simulink model "steeringControlSystemNoFilter"  (R2023b)
settings: Solver=ode4  StartTime=0.0  StopTime=5  FixedStep=0.002  RelTol=1e-3  AbsTol=1e-6  EnableMultiTasking=on
undefined symbols (not defined in the file): den, kd, ki, kp, num, VMAX_DAC
libraries: dspxfrm3 x1
settings Model: ExtModeTrigDuration=10000  Creator=MLevis  LastModifiedBy=JTayl
settings SolverCC: AutoScaleAbsTol=off  AlgebraicLoopSolver=TrustRegion  PositivePriorityOrder=on
settings DataIOCC: SaveFormat=Array  SignalLoggingSaveFormat=ModelDataLogs  ReturnWorkspaceOutputs=off
settings OptimizationCC: BlockReduction=off  BooleanDataType=off  OptimizeBlockIOStorage=off  BufferReuse=off  GlobalBufferReuse=off  ExpressionFolding=off  ExpressionDepthLimit=2147483647  LocalBlockOutputs=off  InitFltsAndDblsToZero=on  LifeSpan=inf  OptimizeDataStoreBuffers=off  BusAssignmentInplaceUpdate=off
settings DebuggingCC: SaveWithParameterizedLinksMsg=none  UnderspecifiedInitializationDetection=Classic  MergeDetectMultiDrivingBlocksExec=none  SignalResolutionControl=TryResolveAllWithWarning  MultiTaskDSMMsg=warning  MultiTaskCondExecSysMsg=none  FcnCallInpInsideContextMsg=warning  UnconnectedInputMsg=warning  UnconnectedOutputMsg=warning  UnconnectedLineMsg=warning  StateNameClashWarn=warning  SFUnexpectedBacktrackingDiag=warning  SFNoUnconditionalDefaultTransitionDiag=warning  SFExecutionAtInitializationDiag=none  ArithmeticOperatorsInVariantConditions=warning
settings HardwareCC: ProdBitPerPointer=32  ProdBitPerSizeT=32  ProdBitPerPtrDiffT=32  ProdLargestAtomicFloat=None  ProdIntDivRoundTo=Undefined  ProdEndianess=Unspecified  ProdWordSize=32  ProdHWDeviceType=32-bit Generic  TargetHWDeviceType=32-bit Generic
settings ModelReferenceCC: EnableRefExpFcnMdlSchedulingChecks=on  PropagateSignalLabelsOutOfModel=off
settings SFSimCC: CustomCodeUndefinedFunction=UseInterfaceOnly
settings RTWCC: Description=Quarc Win32 Target  SystemTargetFile=quarc_windows.tlc  TemplateMakefile=quarc_default_tmf
settings CodeAppCC: StateflowObjectComments=on
settings STFCustomTargetCC: TargetFcnLib=ansi_tfl_tmw.mat  TargetPreCompLibLocation=C:\PROGRA~3\QUARC\lib\2018b\windows\release  TargetLangStandard=C89/C90 (ANSI)  CPPClassGenCompliant=on  GRTInterface=on  SystemTargetFile=quarc_windows.tlc
settings GRTTargetCC: TargetFcnLib=ansi_tfl_tmw.mat  TargetPreCompLibLocation=C:\PROGRA~3\QUARC\lib\2018b\windows\release  TargetLangStandard=C89/C90 (ANSI)  ParMdlRefBuildCompliant=off  CompOptLevelCompliant=off  ConcurrentExecutionCompliant=off  CombineOutputUpdateFcns=off  MatFileLogging=off  GRTInterface=on  UseToolchainInfoCompliant=off  ExtMode=on  ExtModeMexFile=quarc_comm
settings ConfigComp: CovMetricSettings=dw  CovSaveCumulativeToWorkspaceVar=on  CovSaveSingleToWorkspaceVar=on

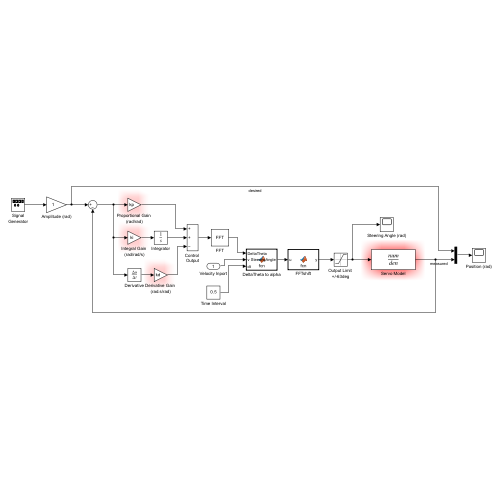
[thumbnail: Simulink's stored preview of the top-level diagram]
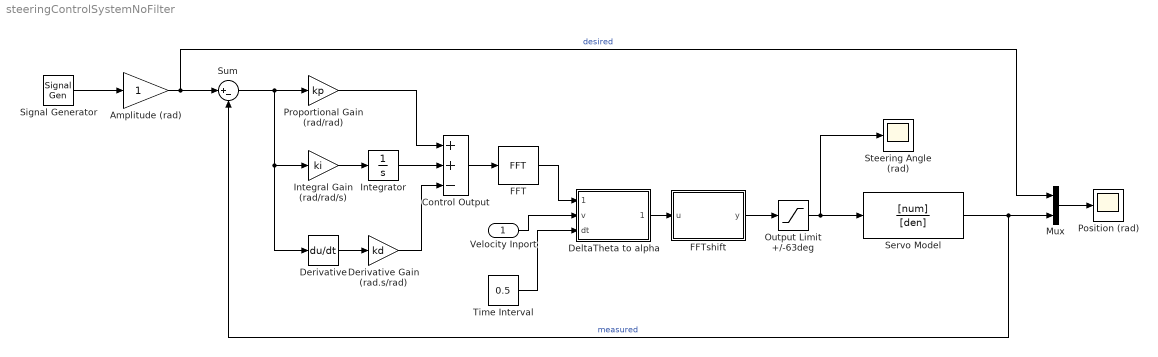
== system steeringControlSystemNoFilter ==
  Velocity Inport : Inport
  Amplitude (rad) : Gain  SaturateOnIntegerOverflow=on  OutDataTypeStr=Inherit: Same as input  ParamDataTypeStr=Inherit: Same as input
  Control Output : Sum  Inputs=++-
  DeltaTheta to alpha : MATLAB Function  TreatAsAtomicUnit=on
  Derivative : Derivative
  Derivative Gain (rad.s/rad) : Gain  Gain=kd
  FFT : dspxfrm3/FFT  FFTImplementation=Auto  CompMethod=Table lookup  TableOpt=NEW  TableOptActive=Speed  BitRevOrder=off  Normalize=off  InheritFFTLength=on  FFTLength=64  WrapInput=on  roundingMode=Floor  overflowMode=off  firstCoeffDataTypeStr=Inherit: Same word length as input  firstCoeffLastDataTypeStr=Inherit: Same word length as input  outputMin=[]  outputMax=[]
  FFTshift : MATLAB Function  TreatAsAtomicUnit=on
  Integral Gain (rad/rad/s) : Gain  Gain=ki
  Integrator : Integrator  UpperSaturationLimit=VMAX_DAC  LowerSaturationLimit=-VMAX_DAC
  Mux : Mux  Inputs=2
  Output Limit +/-63deg : Saturate  UpperLimit=63  LowerLimit=-63
  Position (rad) : Scope
  Proportional Gain (rad/rad) : Gain  Gain=kp
  Servo Model : TransferFcn  Numerator=[num]  Denominator=[den]
  Signal Generator : SignalGenerator  Frequency=0.4  Units=rad/sec
  Steering Angle (rad) : Scope
  Sum : Sum  Inputs=|+-
  Time Interval : Constant  Value=0.5
  wires:
  Mux/1 -> Position (rad)/1
  Signal Generator/1 -> Amplitude (rad)/1
  Amplitude (rad)/1 -> Sum/1, Mux/1  "desired"
  Proportional Gain (rad/rad)/1 -> Control Output/1
  Control Output/1 -> FFT/1
  Integral Gain (rad/rad/s)/1 -> Integrator/1
  Derivative Gain (rad.s/rad)/1 -> Control Output/3
  Integrator/1 -> Control Output/2
  Sum/1 -> Derivative/1, Integral Gain (rad/rad/s)/1, Proportional Gain (rad/rad)/1
  Output Limit +/-63deg/1 -> Steering Angle (rad)/1, Servo Model/1
  Servo Model/1 -> Mux/2, Sum/2  "measured"
  Derivative/1 -> Derivative Gain (rad.s/rad)/1
  FFT/1 -> DeltaTheta to alpha/1(DeltaTheta)
  DeltaTheta to alpha/1(SteeringAngle) -> FFTshift/1(u)
  FFTshift/1(y) -> Output Limit +/-63deg/1
  Time Interval/1 -> DeltaTheta to alpha/3(dt)
  Velocity Inport/1 -> DeltaTheta to alpha/2(v)

== matlab function steeringControlSystemNoFilter/DeltaTheta to alpha ==
  data: DeltaTheta input; SteeringAngle output; v input; dt input
function SteeringAngle  = fcn(DeltaTheta,v,dt)

SteeringAngle = atan2(DeltaTheta*0.515*pi,180*v*dt);

== matlab function steeringControlSystemNoFilter/FFTshift ==
  data: u input; y output
function y = fcn(u)

y = fftshift(u);
